simulink model "ex2_simulink"  (R2023a)
settings: Solver=VariableStepAuto  StartTime=0.0  StopTime=250  RelTol=1e-3
values from neighbouring files (symbols this model uses):
  theta = theta3    (= -90)    [ex2.m]
  Ts = 0.5    [ex2.m]
  xs = 4.1    [ex2.m]
  ys = 0.3    [ex2.m]
libraries: fuzblock x1
settings Model: PacingRate=1.400000  Creator=User  LastModifiedBy=xkoun
settings DataIOCC: ReturnWorkspaceOutputs=off
settings DebuggingCC: UnconnectedInputMsg=warning  UnconnectedOutputMsg=warning  UnconnectedLineMsg=warning
settings ModelReferenceCC: EnableRefExpFcnMdlSchedulingChecks=on
settings RTWCC: DLArmComputeVersion=19.05

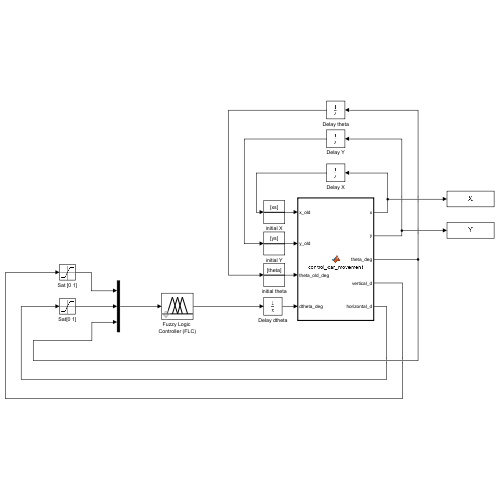
[thumbnail: Simulink's stored preview of the top-level diagram]
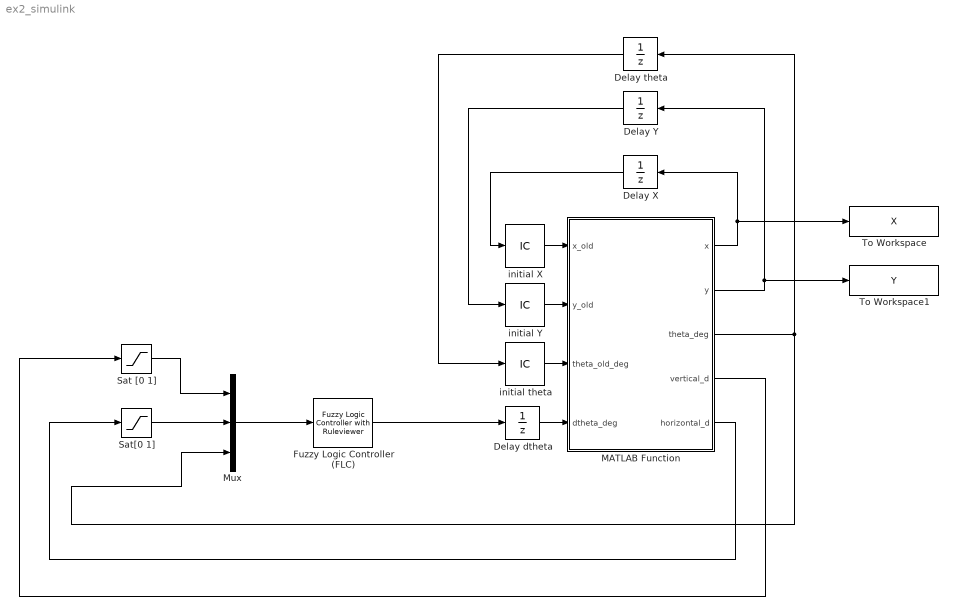
== system ex2_simulink ==
  Delay X : UnitDelay  SampleTime=Ts  HasFrameUpgradeWarning=on
  Delay Y : UnitDelay  SampleTime=Ts  HasFrameUpgradeWarning=on
  Delay dtheta : UnitDelay  SampleTime=Ts  HasFrameUpgradeWarning=on
  Delay theta : UnitDelay  SampleTime=Ts  HasFrameUpgradeWarning=on
  Fuzzy Logic Controller (FLC) : fuzblock/Fuzzy Logic  Controller  with Ruleviewer  fismatrix=car_FLC  Ts=Ts
  MATLAB Function : MATLAB Function  TreatAsAtomicUnit=on
  Mux : Mux  Inputs=3
  Sat [0 1] : Saturate  UpperLimit=1  LowerLimit=0
  Sat[0 1] : Saturate  UpperLimit=1  LowerLimit=0
  To Workspace : ToWorkspace  VariableName=X  SaveFormat=Timeseries  SampleTime=-1
  To Workspace1 : ToWorkspace  VariableName=Y  SaveFormat=Timeseries  SampleTime=-1
  initial X : InitialCondition  Value=xs
  initial Y : InitialCondition  Value=ys
  initial theta : InitialCondition  Value=theta
  wires:
  Delay theta/1 -> initial theta/1
  MATLAB Function/2(y) -> To Workspace1/1, Delay Y/1
  Delay Y/1 -> initial Y/1
  MATLAB Function/1(x) -> To Workspace/1, Delay X/1
  Delay X/1 -> initial X/1
  Fuzzy Logic Controller (FLC)/1 -> Delay dtheta/1
  Mux/1 -> Fuzzy Logic Controller (FLC)/1
  MATLAB Function/4(vertical_d) -> Sat [0 1]/1
  MATLAB Function/5(horizontal_d) -> Sat[0 1]/1
  MATLAB Function/3(theta_deg) -> Mux/3, Delay theta/1
  initial X/1 -> MATLAB Function/1(x_old)
  initial Y/1 -> MATLAB Function/2(y_old)
  initial theta/1 -> MATLAB Function/3(theta_old_deg)
  Sat[0 1]/1 -> Mux/2
  Sat [0 1]/1 -> Mux/1
  Delay dtheta/1 -> MATLAB Function/4(dtheta_deg)

== matlab function ex2_simulink/MATLAB Function ==
  data: x output; x_old input; y output; y_old input; theta_old_deg input; dtheta_deg input; theta_deg output; vertical_d output; horizontal_d output
function [x, y, theta_deg, vertical_d, horizontal_d] = car(x_old, y_old, theta_old_deg, dtheta_deg)
    % Local variables
    if(x_old >= 10)
        u = 0;
    else
        u = 0.05;       % Constant car velocity 
    end
    
    t = 0.5;       % Delay between each calculation
    
    % Calculate the new angle of the car:
    theta_deg = wrapTo180(theta_old_deg + dtheta_deg);
    
    % Calculation of the new position
    x = x_old + u*cosd(theta_deg)*t;
    y = y_old + u*sind(theta_deg)*t;
    
    % ---- horizontal distance to next vertical wall (step wall) ----
    if      y <= 1
        wallX = 5;
    elseif  y <= 2
        wallX = 6;
    elseif  y <= 3 
        wallX = 7;
    else 
        wallX = 20;  % effectively "no wall ahead"
    end
    horizontal_d = max(0, wallX - x);     % clearance (never negative)
    
    % ---- vertical distance to top of current step ----
    if      x <= 5 
        topY = 0;
    elseif  x <= 6 
        topY = 1;
    elseif  x <= 7
        topY = 2;
    else           
        topY = 3;
    end
    vertical_d = max(0, y - topY);      % clearance (never negative)
end
